simulink model "MatPendulum_T3_C_Simulink"  (R2024b)
settings: Solver=VariableStepAuto  StartTime=0.0  StopTime=10.0  RelTol=1e-3
values from neighbouring files (symbols this model uses):
  l = 0.6    [T2_B_T3_C.m]
  m = 0.2038    [T2_B_T3_C.m]
  p = [0, 0, 0]    [T1_B_T3_A.m]    (also in T2_A_T3_B.m = [0, 0]; T2_B_T3_C.m = [0, 1])
settings Model: Creator=lukiq  LastModifiedBy=lukiq

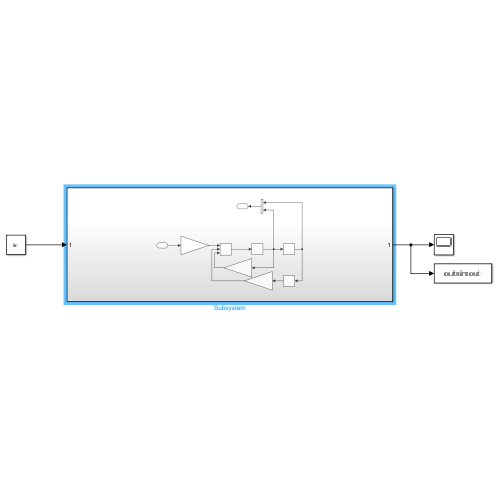
[thumbnail: Simulink's stored preview of the top-level diagram]
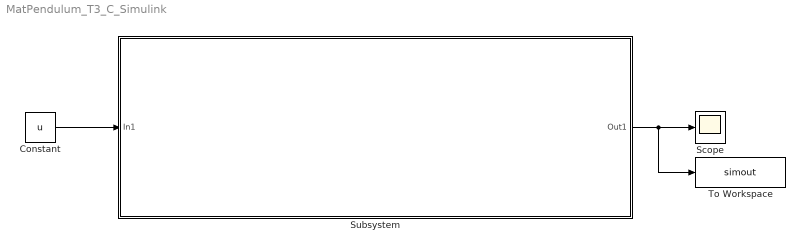
== system MatPendulum_T3_C_Simulink ==
  Constant : Constant  Value=u
  Scope : Scope
  Subsystem : Subsystem
  To Workspace : ToWorkspace  VariableName=simout  SaveFormat=Timeseries  SampleTime=-1
  wires:
  Constant/1 -> Subsystem/1(In1)
  Subsystem/1(Out1) -> To Workspace/1, Scope/1

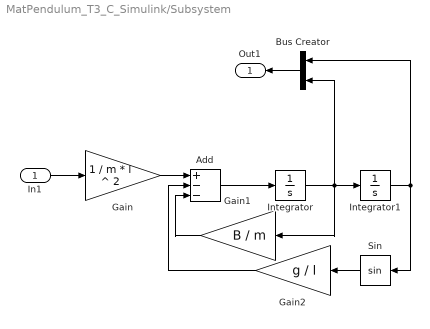
== system MatPendulum_T3_C_Simulink/Subsystem ==
  In1 : Inport
  Add : Sum  Inputs=+--
  Bus Creator : BusCreator  Inputs=2
  Gain : Gain  Gain=1 / m * l ^ 2
  Gain1 : Gain  Gain=B / m
  Gain2 : Gain  Gain=g / l
  Integrator : Integrator  InitialCondition=p(2)
  Integrator1 : Integrator  InitialCondition=p(1)
  Sin : Trigonometry
  Out1 : Outport
  wires:
  Integrator/1 -> Bus Creator/2, Gain1/1, Integrator1/1
  Add/1 -> Integrator/1
  In1/1 -> Gain/1
  Gain/1 -> Add/1
  Gain2/1 -> Add/2
  Integrator1/1 -> Bus Creator/1, Sin/1
  Gain1/1 -> Add/3
  Sin/1 -> Gain2/1
  Bus Creator/1 -> Out1/1
